simulink model "celsioustofernite"  (R2022b)
settings: Solver=VariableStepAuto  StartTime=0.0  StopTime=10.0  RelTol=1e-3
undefined symbols (not defined in the file): x
settings Model: Creator=Brigosha_guest  LastModifiedBy=Brigosha_guest

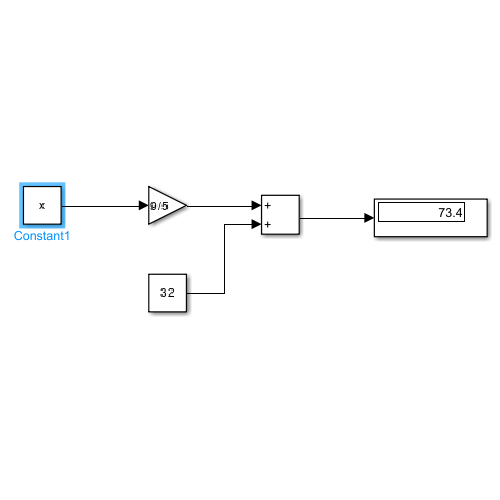
[thumbnail: Simulink's stored preview of the top-level diagram]
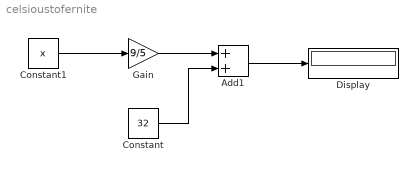
== system celsioustofernite ==
  Add1 : Sum
  Constant : Constant  Value=32
  Constant1 : Constant  Value=x
  Display : Display
  Gain : Gain  Gain=9/5
  wires:
  Gain/1 -> Add1/1
  Constant/1 -> Add1/2
  Add1/1 -> Display/1
  Constant1/1 -> Gain/1
